simulink model "alpha_mod_stimulation"  (R2019a)
settings: Solver=ode3  StartTime=0  StopTime=15  FixedStep=0.002  MaxStep=0.002  RelTol=1e-6  AbsTol=1e-6
libraries: simulink x1
settings Model: ExtModeTrigMode=oneshot  ExtModeArmWhenConnect=off  Creator=suffa  LastModifiedBy=piotr
settings SolverCC: AutoScaleAbsTol=off
settings DataIOCC: SaveFormat=Array  SignalLoggingSaveFormat=ModelDataLogs  SaveOutput=off  SaveTime=off  ReturnWorkspaceOutputs=off
settings OptimizationCC: BlockReduction=off  BooleanDataType=off  ExpressionDepthLimit=2147483647  LifeSpan=inf
settings DebuggingCC: SaveWithParameterizedLinksMsg=none  UnderspecifiedInitializationDetection=Classic  MergeDetectMultiDrivingBlocksExec=none  SignalResolutionControl=TryResolveAllWithWarning  MultiTaskDSMMsg=warning  MultiTaskCondExecSysMsg=none  FcnCallInpInsideContextMsg=warning  StateNameClashWarn=warning  SFUnexpectedBacktrackingDiag=warning  SFNoUnconditionalDefaultTransitionDiag=warning  SFExecutionAtInitializationDiag=none  ArithmeticOperatorsInVariantConditions=warning
settings HardwareCC: ProdBitPerPointer=32  ProdBitPerSizeT=32  ProdBitPerPtrDiffT=32  ProdLargestAtomicFloat=None  ProdIntDivRoundTo=Undefined  ProdEndianess=Unspecified  ProdWordSize=32  ProdHWDeviceType=32-bit Generic  TargetUnknown=on
settings ModelReferenceCC: PropagateSignalLabelsOutOfModel=off
settings SFSimCC: SimUseLocalCustomCode=off
settings RTWCC: TemplateMakefile=grt_vc.tmf  RTWUseLocalCustomCode=off
settings CodeAppCC: StateflowObjectComments=on
settings GRTTargetCC: TargetLangStandard=C89/C90 (ANSI)  GeneratePreprocessorConditionals=Disable all  CombineOutputUpdateFcns=off  GRTInterface=on
settings ConfigComp: CovMetricSettings=dw  CovHtmlReporting=on  CovSaveCumulativeToWorkspaceVar=on  CovSaveSingleToWorkspaceVar=on  CovExternalEMLEnable=off

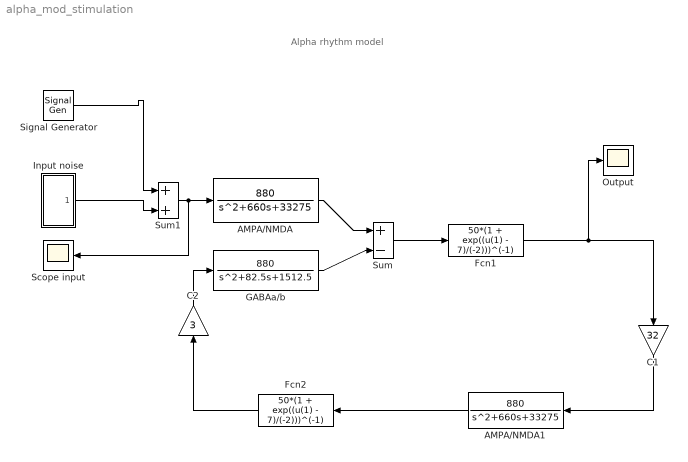
== system alpha_mod_stimulation ==
  note: Alpha rhythm model
  AMPA/NMDA : TransferFcn  Numerator=[880]  Denominator=[1 660 33275]
  AMPA/NMDA1 : TransferFcn  Numerator=[880]  Denominator=[1 660 33275]
  C1 : Gain  Gain=32  SaturateOnIntegerOverflow=on  OutDataTypeStr=Inherit: Same as input  ParamDataTypeStr=Inherit: Same as input
  C2 : Gain  Gain=3  SaturateOnIntegerOverflow=on  OutDataTypeStr=Inherit: Same as input  ParamDataTypeStr=Inherit: Same as input
  Fcn1 : Fcn  Expr=50*(1 + exp((u(1) - 7)/(-2)))^(-1)
  Fcn2 : Fcn  Expr=50*(1 + exp((u(1) - 7)/(-2)))^(-1)
  GABAa/b : TransferFcn  Numerator=[880]  Denominator=[1 82.5 1512.5]
  Input noise : Subsystem
  Output : Scope
  Scope input : Scope
  Signal Generator : SignalGenerator  Amplitude=100  Frequency=5
  Sum : Sum  Inputs=+-  SaturateOnIntegerOverflow=on  InputSameDT=on  OutDataTypeStr=Inherit: Same as first input
  Sum1 : Sum  SaturateOnIntegerOverflow=on  InputSameDT=on  OutDataTypeStr=Inherit: Same as first input
  wires:
  Fcn1/1 -> C1/1, Output/1
  AMPA/NMDA1/1 -> Fcn2/1
  Fcn2/1 -> C2/1
  C2/1 -> GABAa/b/1
  C1/1 -> AMPA/NMDA1/1
  AMPA/NMDA/1 -> Sum/1
  GABAa/b/1 -> Sum/2
  Sum/1 -> Fcn1/1
  Input noise/1(Out1) -> Sum1/2
  Sum1/1 -> AMPA/NMDA/1, Scope input/1
  Signal Generator/1 -> Sum1/1

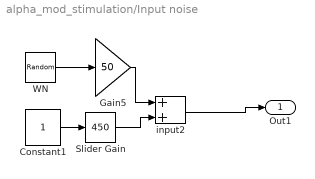
== system alpha_mod_stimulation/Input noise ==
  Constant1 : Constant
  Gain5 : Gain  Gain=50  SaturateOnIntegerOverflow=on  OutDataTypeStr=Inherit: Same as input  ParamDataTypeStr=Inherit: Same as input
  Slider Gain : simulink/Math Operations/Slider Gain  gain=450  low=0  high=700
  WN : RandomNumber  SampleTime=0.002
  input2 : Sum  SaturateOnIntegerOverflow=on  InputSameDT=on  OutDataTypeStr=Inherit: Same as first input
  Out1 : Outport  InitialOutput=0
  wires:
  Constant1/1 -> Slider Gain/1
  Gain5/1 -> input2/1
  WN/1 -> Gain5/1
  Slider Gain/1 -> input2/2
  input2/1 -> Out1/1
